simulink model "body"  (R2017b)
settings: Solver=VariableStepAuto  StartTime=0.0  StopTime=10.0  RelTol=1e-3
settings Model: Creator=Seb  LastModifiedBy=Seb

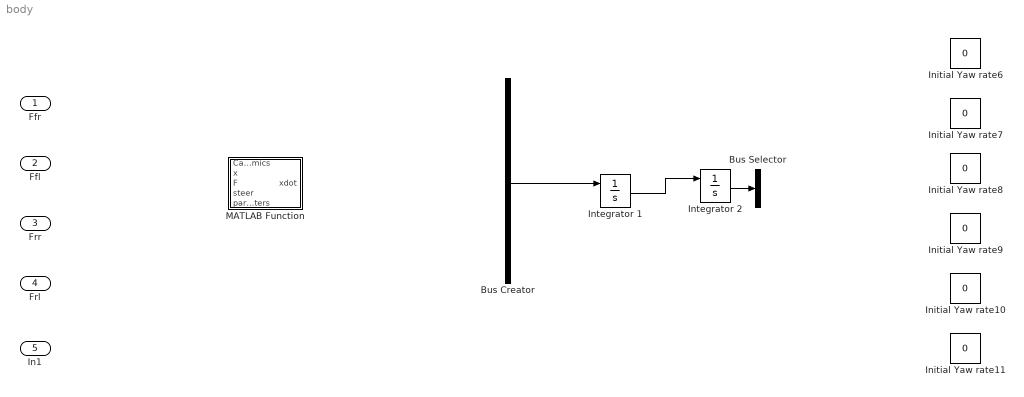
== system body ==
  Ffr : Inport
  Ffl : Inport  Port=2
  Frr : Inport  Port=3
  "Frl " : Inport  Port=4
  In1 : Inport  Port=5
  Bus Selector : BusSelector  OutputSignals=signal1,signal2
  Bus Creator : BusCreator  Inputs=6
  Initial Yaw rate{6..11} (6 alike) : Constant  Value=0
  "Integrator 1 " : Integrator  InitialConditionSource=external
  "Integrator 2 " : Integrator  InitialConditionSource=external
  MATLAB Function : MATLAB Function  TreatAsAtomicUnit=on
  wires:
  Bus Creator/1 -> "Integrator 1 "/1
  "Integrator 1 "/1 -> "Integrator 2 "/1
  "Integrator 2 "/1 -> Bus Selector/1

== matlab function body/MATLAB Function ==
  data: CarDynamics input; xdot output; x input; F input; steer input; parameters input
function xdot = fcn(CarDynamics,x,F,steer,parameters)

xdot = CarDynamics(x,F,steer,parameters);

end
